simulink model "Pendulo2020b"  (R2020b)
settings: Solver=VariableStepAuto  StartTime=0.0  StopTime=100  RelTol=1e-3
values from neighbouring files (symbols this model uses):
  C = 0.0026    [Controlo_PID_Fuzzy.m]
  g = 9.8    [Controlo_PID_Fuzzy.m]
  Jeq = J+m*l^2    (= 0.02128375)    [Controlo_PID_Fuzzy.m]
  l = 0.275    [Controlo_PID_Fuzzy.m]
  m = 0.214    [Controlo_PID_Fuzzy.m]
libraries: fuzblock x1, pid_lib x1
settings Model: Creator=jpmat  LastModifiedBy=jpmat
settings DebuggingCC: UnconnectedInputMsg=none  UnconnectedOutputMsg=none  UnconnectedLineMsg=none
settings ModelReferenceCC: EnableRefExpFcnMdlSchedulingChecks=off

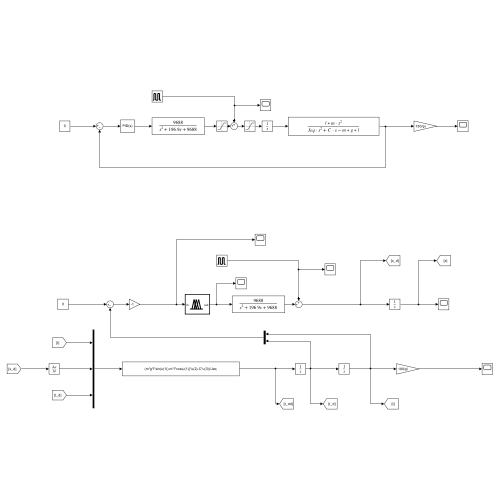
[thumbnail: Simulink's stored preview of the top-level diagram]
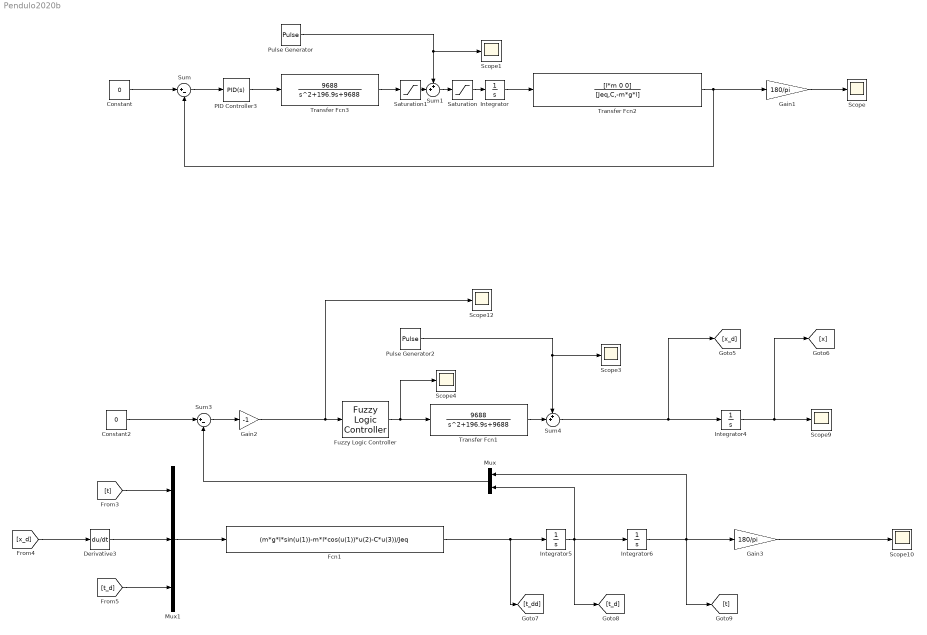
== system Pendulo2020b ==
  Constant : Constant  Value=0
  Constant2 : Constant  Value=0
  Derivative3 : Derivative
  Fcn1 : Fcn  Expr=(m*g*l*sin(u(1))-m*l*cos(u(1))*u(2)-C*u(3))/Jeq
  Fuzzy Logic Controller : fuzblock/Fuzzy Logic  Controller  FIS=pendFIS  OutputSampleNumber=101  DataType=double  FuzzifiedInputs=off  RuleFiringStrengths=off  RuleOutputs=off  AggregatedOutputs=off  SimulateUsing=Interpreted execution  OutOfRangeInputValueMessage=warning  NoRuleFiredMessage=warning  EmptyOutputFuzzySetMessage=warning
  Gain1 : Gain  Gain=180/pi
  Gain2 : Gain  Gain=-1
  Gain3 : Gain  Gain=180/pi
  Integrator{,4..6} (4 alike) : Integrator
  Mux : Mux  Inputs=2
  Mux1 : Mux  Inputs=3
  PID Controller3 : pid_lib/PID Controller  Controller=PID  Form=Parallel  TimeDomain=Continuous-time  UseExternalTs=off  SampleTime=-1  IntegratorMethod=Forward Euler  ControllerParametersSource=internal  P=26.78  I=162.8  D=1.05  N=100  UseFilter=on  TunerSelectOption=Transfer Function Based (PID Tuner App)  InitialConditionSource=internal  InitialConditionForIntegrator=0  InitialConditionForFilter=0  DifferentiatorICPrevScaledInput=0  ExternalReset=none  TrackingMode=off  Kt=1  LimitOutput=off  SatLimitsSource=internal  UpperSaturationLimit=inf  LowerSaturationLimit=-inf  LinearizeAsGain=on  AntiWindupMode=none  Kb=1  POutMin=[]  POutMax=[]  IOutMin=[]  IOutMax=[]  DOutMin=[]  DOutMax=[]  NOutMin=[]  NOutMax=[]  SumOutMin=[]  SumOutMax=[]  SaturationOutMin=[]  SaturationOutMax=[]  PParamMin=[]  PParamMax=[]  IParamMin=[]  IParamMax=[]  DParamMin=[]  DParamMax=[]  NParamMin=[]  NParamMax=[]  KbParamMin=[]  KbParamMax=[]  KtParamMin=[]  KtParamMax=[]  KbOutMin=[]  KbOutMax=[]  KtOutMin=[]  KtOutMax=[]  IntegratorOutMin=[]  IntegratorOutMax=[]  FilterOutMin=[]  FilterOutMax=[]  SumI1OutMin=[]  SumI1OutMax=[]  SumI2OutMin=[]  SumI2OutMax=[]  SumI3OutMin=[]  SumI3OutMax=[]  SumI4OutMin=[]  SumI4OutMax=[]  SumDOutMin=[]  SumDOutMax=[]  DifferentiatorOutMin=[]  DifferentiatorOutMax=[]  FilterDiffOutCoefMin=[]  FilterDiffOutCoefMax=[]  ReciprocalOutMin=[]  ReciprocalOutMax=[]  SumDenOutMin=[]  SumDenOutMax=[]  SumNumOutMin=[]  SumNumOutMax=[]  DivideOutMin=[]  DivideOutMax=[]  UdiffTsProdOutMin=[]  UdiffTsProdOutMax=[]  NTsProdOutMin=[]  NTsProdOutMax=[]  UintegralTsProdOutMin=[]  UintegralTsProdOutMax=[]  UngainTsProdOutMin=[]  UngainTsProdOutMax=[]  IntegratorContinuousStateAttributes=''  IntegratorStateMustResolveToSignalObject=off  IntegratorRTWStateStorageClass=Auto  FilterContinuousStateAttributes=''  FilterStateMustResolveToSignalObject=off  FilterRTWStateStorageClass=Auto  ParallelPVariant=InternalParameters  IdealPVariant=Disabled  IVariant=InternalParameters  DVariant=InternalParameters  IntegratorVariant=Continuous  SatVariant=Disabled  AWVariant=Passthrough  PCopyVariant=Disabled  TRVariant=Disabled  FdbkBlocksVariant=Forward  IdealPFdbkVariant=Disabled  SatFdbkVariant=Disabled  DerivativeFilterVariant=ContFilter  NVariant=InternalParameters  NCopyVariant=Disabled  FilterICVariant=InternalICsFilter  IntegratorICVariant=InternalICs  ExternalResetVariant=Disabled  TRSumVariant=Passthrough  SumFdbkVariant=Disabled  SumVariant=Sum_PID  TsampFilterVariant=InternalTs  TsampNgainVariant=Passthrough  TsampIntegralVariant=Disabled_SignalSpec  ExternalSaturationOutDataTypeStr=Inherit: Same as second input
  Pulse Generator : DiscretePulseGenerator  PulseType=Time based  Amplitude=10  Period=0.5  PulseWidth=5
  Pulse Generator2 : DiscretePulseGenerator  PulseType=Time based  Amplitude=1e-03  Period=0.5  PulseWidth=5
  Saturation : Saturate  UpperLimit=0.3  LowerLimit=-0.3
  Saturation1 : Saturate  UpperLimit=0.3  LowerLimit=-0.3
  Scope{,1,3..4,9..10,12} (7 alike) : Scope
  Sum : Sum  Inputs=|+-
  Sum1 : Sum  Inputs=++|
  Sum3 : Sum  Inputs=|+-
  Sum4 : Sum  Inputs=++|
  Transfer Fcn1 : TransferFcn  Numerator=[9688]  Denominator=[1,196.9,9688]
  Transfer Fcn2 : TransferFcn  Numerator=[l*m 0 0]  Denominator=[Jeq,C,-m*g*l]
  Transfer Fcn3 : TransferFcn  Numerator=[9688]  Denominator=[1,196.9,9688]
  wires:
  Integrator4/1 -> [x], Scope9/1
  Sum4/1 -> [x_d], Integrator4/1
  Transfer Fcn1/1 -> Sum4/2
  Pulse Generator2/1 -> Sum4/1, Scope3/1
  Constant2/1 -> Sum3/1
  Sum3/1 -> Gain2/1
  Gain2/1 -> Fuzzy Logic Controller/1, Scope12/1
  Fuzzy Logic Controller/1 -> Transfer Fcn1/1, Scope4/1
  [x_d] -> Derivative3/1
  Mux1/1 -> Fcn1/1
  [t_d] -> Mux1/3
  Integrator6/1 -> Mux/1, Gain3/1, [t]
  Fcn1/1 -> [t_dd], Integrator5/1
  Integrator5/1 -> Mux/2, [t_d], Integrator6/1
  Derivative3/1 -> Mux1/2
  [t] -> Mux1/1
  Gain3/1 -> Scope10/1
  Saturation/1 -> Integrator/1
  Transfer Fcn3/1 -> Saturation1/1
  Gain1/1 -> Scope/1
  Integrator/1 -> Transfer Fcn2/1
  Transfer Fcn2/1 -> Sum/2, Gain1/1
  Saturation1/1 -> Sum1/2
  Pulse Generator/1 -> Scope1/1, Sum1/1
  Constant/1 -> Sum/1
  Sum1/1 -> Saturation/1
  Sum/1 -> PID Controller3/1
  PID Controller3/1 -> Transfer Fcn3/1
  Mux/1 -> Sum3/2
